simulink model "DT_model_cascade_MHE"  (R2024b)
settings: Solver=VariableStepAuto  StartTime=0.0  StopTime=71  RelTol=1e-4
values from neighbouring files (symbols this model uses):
  E_table = E(V_range2,h_funct(Max_Terminal_V_factor),Sharpness_Const)    [Lookup_Tables.m]    (also in Lookup_Tables_and_Initializer.m)
  P_table = 2 * interp1(PWM,POW,1000+u_range*13)    [Lookup_Tables.m]    (also in Lookup_Tables_and_Initializer.m)
  Q_table = interp1(PWM,NTF,1000+u_range*13)    [DuoCopter_EOM2.m]    (also in Lookup_Tables.m; Lookup_Tables_and_Initializer.m)
  T_table = zeros(size(V_range))    [DuoCopter_EOM2.m]    (also in Lookup_Tables.m; Lookup_Tables_and_Initializer.m)
  u_range = 0:1:100    [DuoCopter_EOM2.m]    (also in Lookup_Tables.m; Lookup_Tables_and_Initializer.m)
  V_range = linspace(0,1.25,10)    [DuoCopter_EOM2.m]    (also in Lookup_Tables.m; Lookup_Tables_and_Initializer.m)
  V_range2 = 0:0.01:1.44    [Lookup_Tables.m]    (also in Lookup_Tables_and_Initializer.m)
undefined symbols (not defined in the file or in its folder): DiscIntNeverNeededParam
libraries: slpidlib x3, simulink x2, eeGeneralControl x1, dspstat3 x1, SignalEditorBlockLib x1
settings Model: Creator=sh2323  LastModifiedBy=sh2323
settings DebuggingCC: AlgebraicLoopMsg=none

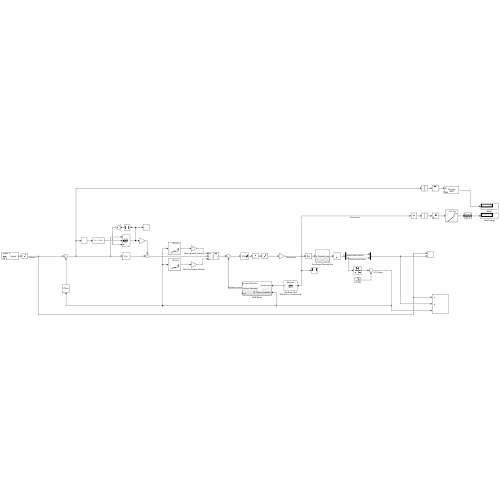
[thumbnail: Simulink's stored preview of the top-level diagram]
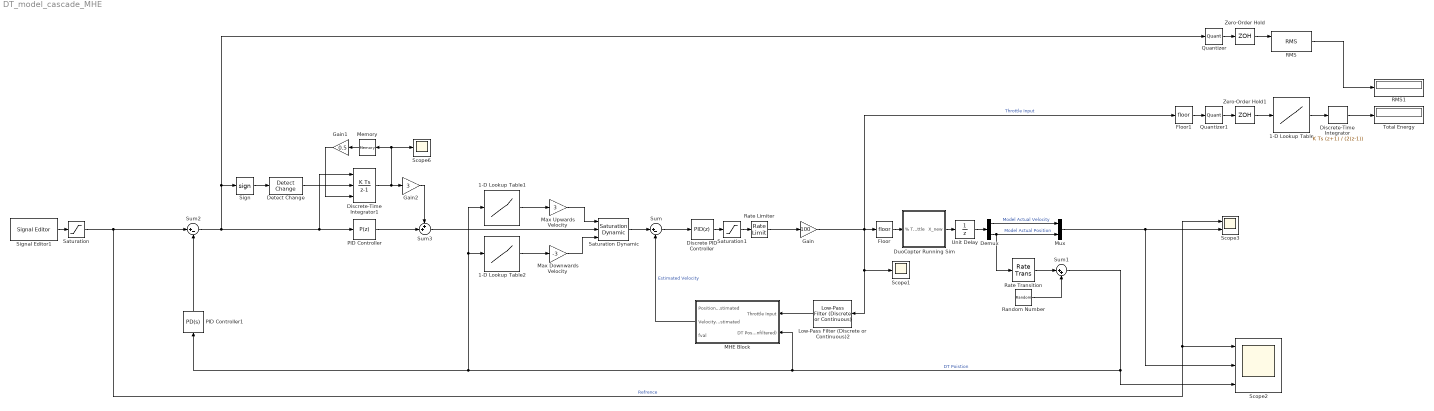
== system DT_model_cascade_MHE ==
  1-D Lookup Table : Lookup_n-D  NumberOfTableDimensions=1  BreakpointsForDimension1=u_range  Table=P_table  InternalRulePriority=Speed  RndMeth=Simplest
  1-D Lookup Table1 : Lookup_n-D  NumberOfTableDimensions=1  BreakpointsForDimension1=V_range2  Table=flip(E_table)  InterpMethod=Nearest  InternalRulePriority=Speed  RndMeth=Simplest
  1-D Lookup Table2 : Lookup_n-D  NumberOfTableDimensions=1  BreakpointsForDimension1=V_range2  Table=E_table  InterpMethod=Nearest  InternalRulePriority=Speed  RndMeth=Simplest
  Demux : Demux  Outputs=2
  Detect Change : simulink/Logic and Bit Operations/Detect Change  vinit=0  OutDataTypeStr=boolean
  Discrete PID Controller : slpidlib/PID Controller  Controller=PID  Form=Parallel  TimeDomain=Discrete-time  UseExternalTs=off  SampleTime=-1  IntegratorMethod=Forward Euler  FilterMethod=Forward Euler  ControllerParametersSource=internal  P=0.2  I=0.05  UseKiTs=off  D=0.1  UseExternalDerivativeSource=off  N=10  UseFilter=on  TunerSelectOption=Transfer Function Based (PID Tuner App)  InitialConditionSource=internal  InitialConditionForIntegrator=0  InitialConditionForFilter=0  DifferentiatorICPrevScaledInput=0  ExternalReset=none  TrackingMode=off  Kt=1  LimitOutput=on  SatLimitsSource=internal  UpperSaturationLimit=1  LowerSaturationLimit=0  LinearizeAsGain=off  AntiWindupMode=none  Kb=1  LimitIntegrator=off  UpperIntegratorSaturationLimit=inf  LowerIntegratorSaturationLimit=-inf  POutMin=[]  POutMax=[]  IOutMin=[]  IOutMax=[]  DOutMin=[]  DOutMax=[]  NOutMin=[]  NOutMax=[]  SumOutMin=[]  SumOutMax=[]  SaturationOutMin=[]  SaturationOutMax=[]  PParamMin=[]  PParamMax=[]  IParamMin=[]  IParamMax=[]  DParamMin=[]  DParamMax=[]  NParamMin=[]  NParamMax=[]  KbParamMin=[]  KbParamMax=[]  KtParamMin=[]  KtParamMax=[]  KbOutMin=[]  KbOutMax=[]  KtOutMin=[]  KtOutMax=[]  IntegratorOutMin=[]  IntegratorOutMax=[]  FilterOutMin=[]  FilterOutMax=[]  SumI1OutMin=[]  SumI1OutMax=[]  SumI2OutMin=[]  SumI2OutMax=[]  SumI3OutMin=[]  SumI3OutMax=[]  SumI4OutMin=[]  SumI4OutMax=[]  SumDOutMin=[]  SumDOutMax=[]  DifferentiatorOutMin=[]  DifferentiatorOutMax=[]  FilterDiffOutCoefMin=[]  FilterDiffOutCoefMax=[]  ReciprocalOutMin=[]  ReciprocalOutMax=[]  SumDenOutMin=[]  SumDenOutMax=[]  SumNumOutMin=[]  SumNumOutMax=[]  DivideOutMin=[]  DivideOutMax=[]  UdiffTsProdOutMin=[]  UdiffTsProdOutMax=[]  NTsProdOutMin=[]  NTsProdOutMax=[]  UintegralTsProdOutMin=[]  UintegralTsProdOutMax=[]  UngainTsProdOutMin=[]  UngainTsProdOutMax=[]  ClampingZeroOutDataTypeStr=Inherit: Inherit via back propagation  ClampingZeroOutMin=[]  ClampingZeroOutMax=[]  FilterDenConstantOutDataTypeStr=Inherit: Inherit via back propagation  FilterDenConstantOutMin=[]  FilterDenConstantOutMax=[]  PCopyOutDataTypeStr=Inherit: Inherit via back propagation  PCopyOutMin=[]  PCopyOutMax=[]  NCopyOutDataTypeStr=Inherit: Inherit via back propagation  NCopyOutMin=[]  NCopyOutMax=[]  IntegratorContinuousStateAttributes=''  IntegratorStateMustResolveToSignalObject=off  IntegratorRTWStateStorageClass=Auto  FilterContinuousStateAttributes=''  FilterStateMustResolveToSignalObject=off  FilterRTWStateStorageClass=Auto  ParallelPVariant=InternalParameters  IdealPVariant=Disabled  IVariant=InternalParameters  DVariant=InternalParameters  IntegratorVariant=Discrete  SatVariant=Enabled  AWVariant=Passthrough  PCopyVariant=Disabled  TRVariant=Disabled  FdbkBlocksVariant=Forward  IdealPFdbkVariant=Disabled  SatFdbkVariant=Disabled  DerivativeFilterVariant=ForwardEulerFilter  NVariant=InternalParameters  NCopyVariant=Disabled  FilterICVariant=InternalICsFilter  IntegratorICVariant=InternalICs  ExternalResetVariant=Disabled  TRSumVariant=Passthrough  SumFdbkVariant=Disabled  SumVariant=Sum_PID  TsampFilterVariant=InternalTs  TsampNgainVariant=Passthrough  TsampIntegralVariant=Disabled_SignalSpec  ExternalSaturationOutDataTypeStr=Inherit: Same as second input  DerivativeSourceVariant=ErrorSignal  PreIntVariant=InternalPreInt
      settings: LibrarySourceBlock=simulink/Discrete/Discrete PID Controller
  Discrete-Time Integrator : DiscreteIntegrator  IntegratorMethod=Integration: Trapezoidal  SampleTime=-1  ICPrevOutput=DiscIntNeverNeededParam  ICPrevScaledInput=DiscIntNeverNeededParam
  Discrete-Time Integrator1 : DiscreteIntegrator  ExternalReset=level  InitialConditionSource=external  SampleTime=-1  ICPrevOutput=DiscIntNeverNeededParam  ICPrevScaledInput=DiscIntNeverNeededParam
  DuoCopter Running Sim : Subsystem
  Floor : Rounding
  Floor1 : Rounding
  Gain : Gain  Gain=100
  Gain1 : Gain  Gain=0.5
  Gain2 : Gain  Gain=3
  Low-Pass Filter (Discrete or Continuous)2 : eeGeneralControl/Low-Pass Filter (Discrete or Continuous)  K=1  T=5  B=inf  A=-inf  init_option=Inherited from block input  x0=0  Ts=-1
  MHE Block : Subsystem
  Max Downwards Velocity : Gain  Gain=-3
  Max Upwards Velocity : Gain  Gain=3
  Memory : Memory
  Mux : Mux  Inputs=2
  PID Controller : slpidlib/PID Controller  Controller=P  Form=Parallel  TimeDomain=Discrete-time  UseExternalTs=off  SampleTime=-1  IntegratorMethod=Forward Euler  FilterMethod=Forward Euler  ControllerParametersSource=internal  P=2  I=4  UseKiTs=off  D=0  UseExternalDerivativeSource=off  N=10  UseFilter=on  TunerSelectOption=Transfer Function Based (PID Tuner App)  InitialConditionSource=internal  InitialConditionForIntegrator=0  InitialConditionForFilter=0  DifferentiatorICPrevScaledInput=0  ExternalReset=none  TrackingMode=off  Kt=1  LimitOutput=off  SatLimitsSource=internal  UpperSaturationLimit=inf  LowerSaturationLimit=-inf  LinearizeAsGain=on  AntiWindupMode=none  Kb=1  LimitIntegrator=off  UpperIntegratorSaturationLimit=inf  LowerIntegratorSaturationLimit=-inf  POutMin=[]  POutMax=[]  IOutMin=[]  IOutMax=[]  DOutMin=[]  DOutMax=[]  NOutMin=[]  NOutMax=[]  SumOutMin=[]  SumOutMax=[]  SaturationOutMin=[]  SaturationOutMax=[]  PParamMin=[]  PParamMax=[]  IParamMin=[]  IParamMax=[]  DParamMin=[]  DParamMax=[]  NParamMin=[]  NParamMax=[]  KbParamMin=[]  KbParamMax=[]  KtParamMin=[]  KtParamMax=[]  KbOutMin=[]  KbOutMax=[]  KtOutMin=[]  KtOutMax=[]  IntegratorOutMin=[]  IntegratorOutMax=[]  FilterOutMin=[]  FilterOutMax=[]  SumI1OutMin=[]  SumI1OutMax=[]  SumI2OutMin=[]  SumI2OutMax=[]  SumI3OutMin=[]  SumI3OutMax=[]  SumI4OutMin=[]  SumI4OutMax=[]  SumDOutMin=[]  SumDOutMax=[]  DifferentiatorOutMin=[]  DifferentiatorOutMax=[]  FilterDiffOutCoefMin=[]  FilterDiffOutCoefMax=[]  ReciprocalOutMin=[]  ReciprocalOutMax=[]  SumDenOutMin=[]  SumDenOutMax=[]  SumNumOutMin=[]  SumNumOutMax=[]  DivideOutMin=[]  DivideOutMax=[]  UdiffTsProdOutMin=[]  UdiffTsProdOutMax=[]  NTsProdOutMin=[]  NTsProdOutMax=[]  UintegralTsProdOutMin=[]  UintegralTsProdOutMax=[]  UngainTsProdOutMin=[]  UngainTsProdOutMax=[]  ClampingZeroOutDataTypeStr=Inherit: Inherit via back propagation  ClampingZeroOutMin=[]  ClampingZeroOutMax=[]  FilterDenConstantOutDataTypeStr=Inherit: Inherit via back propagation  FilterDenConstantOutMin=[]  FilterDenConstantOutMax=[]  PCopyOutDataTypeStr=Inherit: Inherit via back propagation  PCopyOutMin=[]  PCopyOutMax=[]  NCopyOutDataTypeStr=Inherit: Inherit via back propagation  NCopyOutMin=[]  NCopyOutMax=[]  IntegratorContinuousStateAttributes=''  IntegratorStateMustResolveToSignalObject=off  IntegratorRTWStateStorageClass=Auto  FilterContinuousStateAttributes=''  FilterStateMustResolveToSignalObject=off  FilterRTWStateStorageClass=Auto  ParallelPVariant=InternalParameters  IdealPVariant=Disabled  IVariant=Disabled  DVariant=Disabled  IntegratorVariant=Disabled  SatVariant=Disabled  AWVariant=Disabled  PCopyVariant=Disabled  TRVariant=Disabled  FdbkBlocksVariant=Forward  IdealPFdbkVariant=Disabled  SatFdbkVariant=Disabled  DerivativeFilterVariant=Disabled  NVariant=Disabled  NCopyVariant=Disabled_SignalSpec  FilterICVariant=Disabled  IntegratorICVariant=Disabled  ExternalResetVariant=Disabled  TRSumVariant=Passthrough  SumFdbkVariant=Disabled  SumVariant=Passthrough_P  TsampFilterVariant=InternalTs  TsampNgainVariant=Passthrough  TsampIntegralVariant=Disabled_SignalSpec  ExternalSaturationOutDataTypeStr=Inherit: Same as second input  DerivativeSourceVariant=Disabled  PreIntVariant=InternalPreInt
  PID Controller1 : slpidlib/PID Controller  Controller=PD  Form=Parallel  TimeDomain=Continuous-time  UseExternalTs=off  SampleTime=-1  IntegratorMethod=Forward Euler  FilterMethod=Forward Euler  ControllerParametersSource=internal  P=1  I=1  UseKiTs=off  D=0.075  UseExternalDerivativeSource=off  N=10  UseFilter=on  TunerSelectOption=Transfer Function Based (PID Tuner App)  InitialConditionSource=internal  InitialConditionForIntegrator=0  InitialConditionForFilter=0  DifferentiatorICPrevScaledInput=0  ExternalReset=none  TrackingMode=off  Kt=1  LimitOutput=off  SatLimitsSource=internal  UpperSaturationLimit=inf  LowerSaturationLimit=-inf  LinearizeAsGain=on  AntiWindupMode=none  Kb=1  LimitIntegrator=off  UpperIntegratorSaturationLimit=inf  LowerIntegratorSaturationLimit=-inf  POutMin=[]  POutMax=[]  IOutMin=[]  IOutMax=[]  DOutMin=[]  DOutMax=[]  NOutMin=[]  NOutMax=[]  SumOutMin=[]  SumOutMax=[]  SaturationOutMin=[]  SaturationOutMax=[]  PParamMin=[]  PParamMax=[]  IParamMin=[]  IParamMax=[]  DParamMin=[]  DParamMax=[]  NParamMin=[]  NParamMax=[]  KbParamMin=[]  KbParamMax=[]  KtParamMin=[]  KtParamMax=[]  KbOutMin=[]  KbOutMax=[]  KtOutMin=[]  KtOutMax=[]  IntegratorOutMin=[]  IntegratorOutMax=[]  FilterOutMin=[]  FilterOutMax=[]  SumI1OutMin=[]  SumI1OutMax=[]  SumI2OutMin=[]  SumI2OutMax=[]  SumI3OutMin=[]  SumI3OutMax=[]  SumI4OutMin=[]  SumI4OutMax=[]  SumDOutMin=[]  SumDOutMax=[]  DifferentiatorOutMin=[]  DifferentiatorOutMax=[]  FilterDiffOutCoefMin=[]  FilterDiffOutCoefMax=[]  ReciprocalOutMin=[]  ReciprocalOutMax=[]  SumDenOutMin=[]  SumDenOutMax=[]  SumNumOutMin=[]  SumNumOutMax=[]  DivideOutMin=[]  DivideOutMax=[]  UdiffTsProdOutMin=[]  UdiffTsProdOutMax=[]  NTsProdOutMin=[]  NTsProdOutMax=[]  UintegralTsProdOutMin=[]  UintegralTsProdOutMax=[]  UngainTsProdOutMin=[]  UngainTsProdOutMax=[]  ClampingZeroOutDataTypeStr=Inherit: Inherit via back propagation  ClampingZeroOutMin=[]  ClampingZeroOutMax=[]  FilterDenConstantOutDataTypeStr=Inherit: Inherit via back propagation  FilterDenConstantOutMin=[]  FilterDenConstantOutMax=[]  PCopyOutDataTypeStr=Inherit: Inherit via back propagation  PCopyOutMin=[]  PCopyOutMax=[]  NCopyOutDataTypeStr=Inherit: Inherit via back propagation  NCopyOutMin=[]  NCopyOutMax=[]  IntegratorContinuousStateAttributes=''  IntegratorStateMustResolveToSignalObject=off  IntegratorRTWStateStorageClass=Auto  FilterContinuousStateAttributes=''  FilterStateMustResolveToSignalObject=off  FilterRTWStateStorageClass=Auto  ParallelPVariant=InternalParameters  IdealPVariant=Disabled  IVariant=Disabled  DVariant=InternalParameters  IntegratorVariant=Disabled  SatVariant=Disabled  AWVariant=Disabled  PCopyVariant=Disabled  TRVariant=Disabled  FdbkBlocksVariant=Forward  IdealPFdbkVariant=Disabled  SatFdbkVariant=Disabled  DerivativeFilterVariant=ContFilter  NVariant=InternalParameters  NCopyVariant=Disabled  FilterICVariant=InternalICsFilter  IntegratorICVariant=Disabled  ExternalResetVariant=Disabled  TRSumVariant=Passthrough  SumFdbkVariant=Disabled  SumVariant=Sum_PD  TsampFilterVariant=InternalTs  TsampNgainVariant=Passthrough  TsampIntegralVariant=Disabled_SignalSpec  ExternalSaturationOutDataTypeStr=Inherit: Same as second input  DerivativeSourceVariant=ErrorSignal  PreIntVariant=InternalPreInt
  Quantizer : Quantizer  QuantizationInterval=0.05
  Quantizer1 : Quantizer  QuantizationInterval=0.05
  RMS : dspstat3/RMS  run=on  directionMode=Each column  dimension=1  reset_popup=Non-zero sample
  RMS1 : Display
  Random Number : RandomNumber  Variance=0.0001  SampleTime=0.05
  Rate Limiter : RateLimiter  RisingSlewLimit=8  FallingSlewLimit=-10  SampleTimeMode=inherited
  Rate Transition : RateTransition  OutPortSampleTime=0.05
  Saturation : Saturate  UpperLimit=1.44  LowerLimit=0
  Saturation Dynamic : simulink/Discontinuities/Saturation Dynamic  OutMin=[]  OutMax=[]  OutDataTypeStr=Inherit: Same as second input  OutDataType=fixdt(1, 16)  OutScaling=2^-10  DoSatur=off
  Saturation1 : Saturate  UpperLimit=0.9  LowerLimit=0
  Scope1 : Scope
  Scope2 : Scope  NumInputPorts=3
  Scope3 : Scope  NumInputPorts=2
  Scope6 : Scope
  Sign : Signum
  Signal Editor1 : SignalEditorBlockLib/Signal Editor  FileName=samplemission.mat  ActiveScenario=Scenario  ActiveSignal=Signal 1  IsBus=off  OutputBusObjectStr=Bus: BusObject  SampleTime=0  ZeroCross=off  OutputAfterFinalValue=Setting to zero  Unit=inherit  PreserveSignalName=on  ApplySigPropsToAllScenarios=on  ApplySigPropsToAllSignals=off
  Sum : Sum  Inputs=|+-
  Sum1 : Sum  Inputs=|++
  Sum2 : Sum  Inputs=|+-
  Sum3 : Sum  Inputs=++|
  Total Energy : Display
  Unit Delay : UnitDelay  SampleTime=-1  HasFrameUpgradeWarning=on
  Zero-Order Hold : ZeroOrderHold  SampleTime=-1
  Zero-Order Hold1 : ZeroOrderHold  SampleTime=-1
  wires:
  Demux/1 -> Mux/1  "Model Actual Velocity"
  Demux/2 -> Mux/2, Rate Transition/1  "Model Actual Position"
  Discrete PID Controller/1 -> Saturation1/1
  Signal Editor1/1 -> Saturation/1
  Saturation1/1 -> Rate Limiter/1
  Rate Limiter/1 -> Gain/1
  DuoCopter Running Sim/1(X_new) -> Unit Delay/1
  Unit Delay/1 -> Demux/1
  Rate Transition/1 -> Sum1/1
  Random Number/1 -> Sum1/2
  Sum1/1 -> Scope2/3, PID Controller1/1, 1-D Lookup Table1/1, 1-D Lookup Table2/1, MHE Block/2(DT Position (Unfiltered))  "DT Poistion"
  Saturation/1 -> Scope3/1, Scope2/1, Sum2/1  "Refrence"
  MHE Block/2(Velocity Estimated) -> Sum/2  "Estimated Velocity"
  Low-Pass Filter (Discrete or Continuous)2/1 -> MHE Block/1(Throttle Input)
  Quantizer1/1 -> Zero-Order Hold1/1
  Zero-Order Hold1/1 -> 1-D Lookup Table/1
  Gain/1 -> Floor/1, Floor1/1, Low-Pass Filter (Discrete or Continuous)2/1, Scope1/1  "Throttle Input"
  1-D Lookup Table/1 -> Discrete-Time Integrator/1
  Discrete-Time Integrator/1 -> Total Energy/1
  RMS/1 -> RMS1/1
  Zero-Order Hold/1 -> RMS/1
  Quantizer/1 -> Zero-Order Hold/1
  Sum/1 -> Discrete PID Controller/1
  Saturation Dynamic/1 -> Sum/1
  1-D Lookup Table1/1 -> Max Upwards Velocity/1
  1-D Lookup Table2/1 -> Max Downwards Velocity/1
  Max Upwards Velocity/1 -> Saturation Dynamic/1
  Max Downwards Velocity/1 -> Saturation Dynamic/3
  Floor/1 -> DuoCopter Running Sim/1(% Throttle)
  Floor1/1 -> Quantizer1/1
  Mux/1 -> Scope3/2, Scope2/2
  Gain2/1 -> Sum3/1
  Detect Change/1 -> Discrete-Time Integrator1/2
  Gain1/1 -> Discrete-Time Integrator1/3
  Memory/1 -> Gain1/1
  Sign/1 -> Detect Change/1
  Sum2/1 -> PID Controller/1, Discrete-Time Integrator1/1, Quantizer/1, Sign/1
  Discrete-Time Integrator1/1 -> Memory/1, Scope6/1, Gain2/1
  PID Controller/1 -> Sum3/2
  Sum3/1 -> Saturation Dynamic/2
  PID Controller1/1 -> Sum2/2

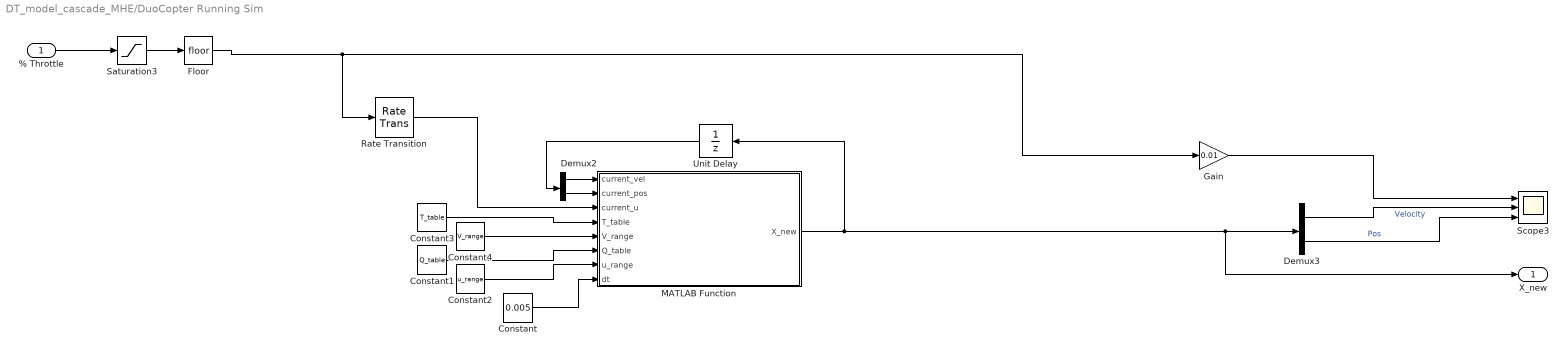
== system DT_model_cascade_MHE/DuoCopter Running Sim ==
  % Throttle : Inport
  Constant : Constant  Value=0.005
  Constant1 : Constant  Value=Q_table
  Constant2 : Constant  Value=u_range
  Constant3 : Constant  Value=T_table
  Constant4 : Constant  Value=V_range
  Demux2 : Demux  Outputs=2
  Demux3 : Demux  Outputs=2
  Floor : Rounding
  Gain : Gain  Gain=0.01
  MATLAB Function : MATLAB Function  TreatAsAtomicUnit=on
  Rate Transition : RateTransition  OutPortSampleTime=0.005
  Saturation3 : Saturate  UpperLimit=100  LowerLimit=0
  Scope3 : Scope  NumInputPorts=3
  Unit Delay : UnitDelay  SampleTime=-1  HasFrameUpgradeWarning=on
  X_new : Outport
  wires:
  % Throttle/1 -> Saturation3/1
  Saturation3/1 -> Floor/1
  Floor/1 -> Gain/1, Rate Transition/1
  Constant/1 -> MATLAB Function/8(dt)
  Constant1/1 -> MATLAB Function/6(Q_table)
  Constant2/1 -> MATLAB Function/7(u_range)
  Demux2/2 -> MATLAB Function/2(current_pos)
  Demux2/1 -> MATLAB Function/1(current_vel)
  Constant3/1 -> MATLAB Function/4(T_table)
  Constant4/1 -> MATLAB Function/5(V_range)
  Rate Transition/1 -> MATLAB Function/3(current_u)
  Demux3/1 -> Scope3/2  "Velocity"
  Demux3/2 -> Scope3/3  "Pos"
  MATLAB Function/1(X_new) -> Unit Delay/1, Demux3/1, X_new/1
  Unit Delay/1 -> Demux2/1
  Gain/1 -> Scope3/1

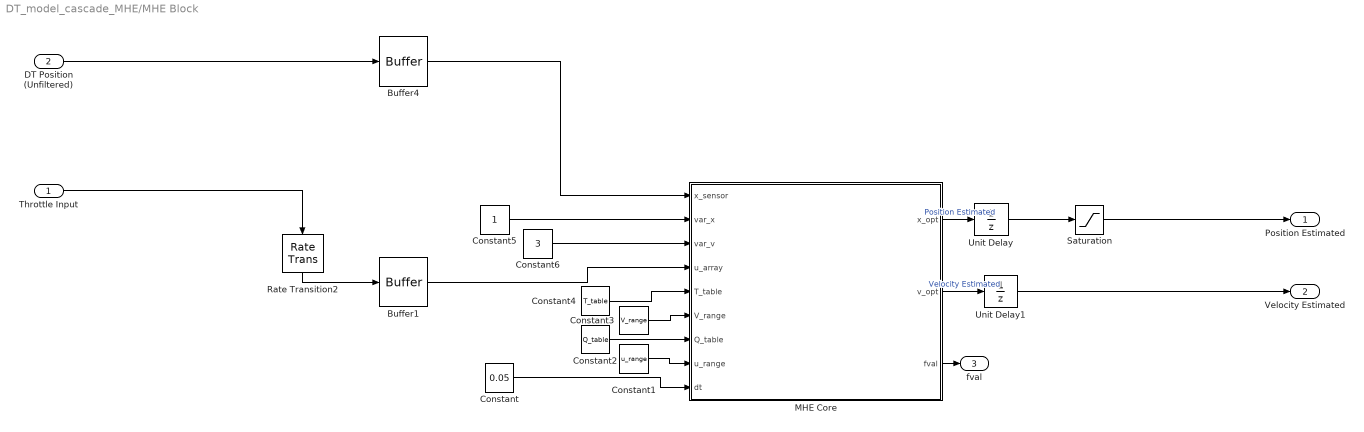
== system DT_model_cascade_MHE/MHE Block ==
  Throttle Input : Inport
  DT Position (Unfiltered) : Inport  Port=2
  Buffer1 : Buffer  N=6  V=5  OutputFrames=off
  Buffer4 : Buffer  N=6  V=5  OutputFrames=off
  Constant : Constant  Value=0.05
  Constant1 : Constant  Value=u_range
  Constant2 : Constant  Value=Q_table
  Constant3 : Constant  Value=V_range
  Constant4 : Constant  Value=T_table
  Constant5 : Constant
  Constant6 : Constant  Value=3
  MHE Core : MATLAB Function  TreatAsAtomicUnit=on
  Rate Transition2 : RateTransition  OutPortSampleTime=0.05
  Saturation : Saturate  UpperLimit=1.44  LowerLimit=0
  Unit Delay : UnitDelay  SampleTime=-1  HasFrameUpgradeWarning=on
  Unit Delay1 : UnitDelay  SampleTime=-1  HasFrameUpgradeWarning=on
  Position Estimated : Outport
  Velocity Estimated : Outport  Port=2
  fval : Outport  Port=3
  wires:
  Constant2/1 -> MHE Core/7(Q_table)
  Rate Transition2/1 -> Buffer1/1
  Constant4/1 -> MHE Core/5(T_table)
  Constant1/1 -> MHE Core/8(u_range)
  Constant6/1 -> MHE Core/3(var_v)
  Constant/1 -> MHE Core/9(dt)
  Constant5/1 -> MHE Core/2(var_x)
  Constant3/1 -> MHE Core/6(V_range)
  Buffer4/1 -> MHE Core/1(x_sensor)
  Buffer1/1 -> MHE Core/4(u_array)
  MHE Core/2(v_opt) -> Unit Delay1/1  "Velocity Estimated"
  DT Position (Unfiltered)/1 -> Buffer4/1
  Throttle Input/1 -> Rate Transition2/1
  MHE Core/3(fval) -> fval/1
  MHE Core/1(x_opt) -> Unit Delay/1  "Position Estimated"
  Saturation/1 -> Position Estimated/1
  Unit Delay/1 -> Saturation/1
  Unit Delay1/1 -> Velocity Estimated/1

== matlab function DT_model_cascade_MHE/DuoCopter Running Sim/MATLAB Function ==
  data: current_vel input; X_new output; current_pos input; current_u input; T_table input; V_range input; Q_table input; u_range input; dt input
function X_new = DT_EOM_fcn2(current_vel,current_pos,current_u,T_table,V_range,Q_table,u_range,dt)

X_current = [current_vel;current_pos];
%% System Parameters

% Constants
g = 9.81;
mu = 1; % mu ranges from 0.11 to 0.17

% Motor choice
m_prop = 0.006;
m_motor = 0.076;
m_esc = 0.042;
m_des = 0.200;
m_cw = 0.400;

% Rail Constraints
x_bottom = 0;
x_top = 1.44;

% Total cart mass (cart mass + arm + propellers + motors + ESC)
m_c = 0.55 + m_des + m_prop + m_motor + m_esc;

% Inertial Mass (cart+counterwieght)
m_i = m_c + m_cw;

% Length dimensions
l_T = 0.045;
l_g = 0.085;
l_c = 0.055;
h = 0.2104;

%% Key Functions

Q = interp1(u_range,Q_table,current_u,"nearest",'extrap');
T = interp1(V_range,T_table,current_pos,"nearest",'extrap');

% Friction Force Function  (N)
F = @(Q,T) abs(2*Q*l_g - g*m_c*l_c - 2*T*l_T )*(mu/h) ;
% Non-Fricative Forces (N)
N = @(Q,T) 2.*Q - 2.*T - (m_c-m_cw)*g ;
% Static Friction Force (N)
ST = 1.3;

%% Equations of Motion

% X_current(1) ---> Velocity at n
% X_current(2) ---> Position at n

% X_new(1) ---> Velocity at n+1
% X_new(2) ---> Position at n+1

X_new = zeros(2,1);

% static tolerance

tol = 0.001;
edge_tol = 0.001;

% acceleration at either bound must only be in a specific direction
    % if velocity is greater than 0+tol. , friction acts downwards
    % if velocity is less than 0-tol. friction acts upwards
    % if velocity is within the 'static' range:
        % if non-fricative forces are greater than static force, accel nonzero
        % if non-fricative forces are less than static, accel is zero




if  (X_current(1) >= -tol) && (X_current(1) <= tol)

     if abs(N(Q,T)) < ST
        % If non-fricative force can't overcome static friction, no accel
        X_new(1) = 0;
     elseif N(Q,T) > ST
        % Starting upwards, downwards friction
        X_new(1) = X_current(1) + dt*( N(Q,T) - ST )/m_i;
     elseif N(Q,T) < -ST
        % Starting upwards, downwards friction
        X_new(1) = X_current(1) + dt*( N(Q,T) + ST )/m_i;
     end

elseif X_current(1) > tol
    % Moving Upwards, Downwards Friction
    X_new(1) = X_current(1) + dt*( N(Q,T) - F(Q,T) )/m_i;

elseif X_current(1) < -tol
    % Moving Downwards, Upwards Friction
    X_new(1) = X_current(1) + dt*( N(Q,T) + F(Q,T) )/m_i;
end

% Position State Updates
X_new(2) = X_current(2) + dt * 0.5 * (X_current(1) + X_new(1));

%% Edge Impacts

% if located at the top, velocity must be zero or negative
% if locatede at the bottom, velocity must be zero or positive


if X_current(2) >= x_top-edge_tol
    if X_new(1) >= 0
        X_new(1) = 0;
    end
    if X_new(2) > x_top
        X_new(2) = x_top;
    end
elseif X_current(2) <= x_bottom+edge_tol
    if X_new(1) <= 0
        X_new(1) = 0;
    end
    if X_new(2) < x_bottom
        X_new(2) = x_bottom;
    end
end


if X_new(2) > x_top
        X_new(2) = x_top;
elseif X_new(2) < x_bottom
        X_new(2) = x_bottom;
end

== matlab function DT_model_cascade_MHE/MHE Block/MHE Core ==
  data: x_sensor input size=[6,1]; x_opt output double size=1; var_x input; var_v input; u_array input; T_table input; V_range input; Q_table input; u_range input; dt input; v_opt output double size=1; fval output
function [x_opt, v_opt, fval] = nonlinear_estimator3(x_sensor, var_x, var_v, u_array, T_table, V_range, Q_table, u_range, dt)
    n = length(x_sensor);
    
    x_sensor = x_sensor';
    u_array = u_array';


    % Dynamics function (vectorized)
    h = @(v,x,u) DT_EOM_fcn2(v, x, u, T_table, V_range, Q_table, u_range, dt);
    
    % Initial guess (smoothed velocity)

    v_init = diff(x_sensor) / dt;
    v_init = [v_init, v_init(end)]'; % pad last element to length n

    z0 = [v_init; x_sensor(:)];
    
    % Objective function (weighted residuals)
    objfun = @(z) ...
        sum( (x_sensor - z(n+1:end)').^2 / var_x ) + ...  % Measurement residuals
        sum( (z(2:n) - z(1:n-1) ).^2 / var_v );          % Velocity smoothness
    
    % Nonlinear constraints: Enforce dynamics
    nonlcon = @(z) dynamics_constraints(z, n, u_array, h);
    
    % Solver options
    options = optimoptions('fmincon', 'Display', 'iter', 'Algorithm', 'sqp');
    
    % Solve MHE
    [z_opt, fval] = fmincon(objfun, z0, [], [], [], [], [], [], nonlcon, options);
    
    % Extract estimates
    %v_opt = z_opt(1:n);
    %x_opt = z_opt(n+1:end);

    
    v_opt = z_opt(n);
    x_opt = z_opt(end);
end

% Nonlinear constraints to enforce dynamics
function [c, ceq] = dynamics_constraints(z, n, u_array, h)
    v = z(1:n);
    x = z(n+1:end);
    ceq = zeros(2*(n-1), 1);  % Equality constraints
    
    for i = 1:n-1
        % Predict next state using DT_EOM_fcn2
        x_next = h(v(i), x(i), u_array(i));
        
        % Enforce v_next and x_next match dynamics
        ceq(2*i-1) = v(i+1) - x_next(1);  % Velocity constraint
        ceq(2*i)   = x(i+1) - x_next(2);  % Position constraint
    end
    
    c = [];  % No inequality constraints
end
